simulink model "swhl_arch"  (R2024a)
settings: Solver=FixedStepDiscrete  StartTime=0.0  StopTime=10.0  RelTol=1e-3
undefined symbols (not defined in the file or in its folder): D1, P
settings Model: Creator=Inquisitor  LastModifiedBy=Inquisitor

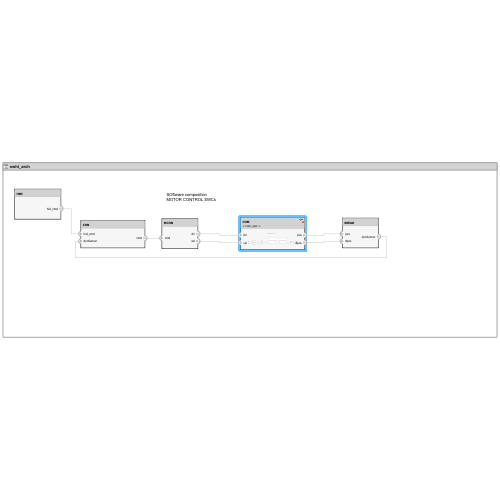
[thumbnail: Simulink's stored preview of the top-level diagram]
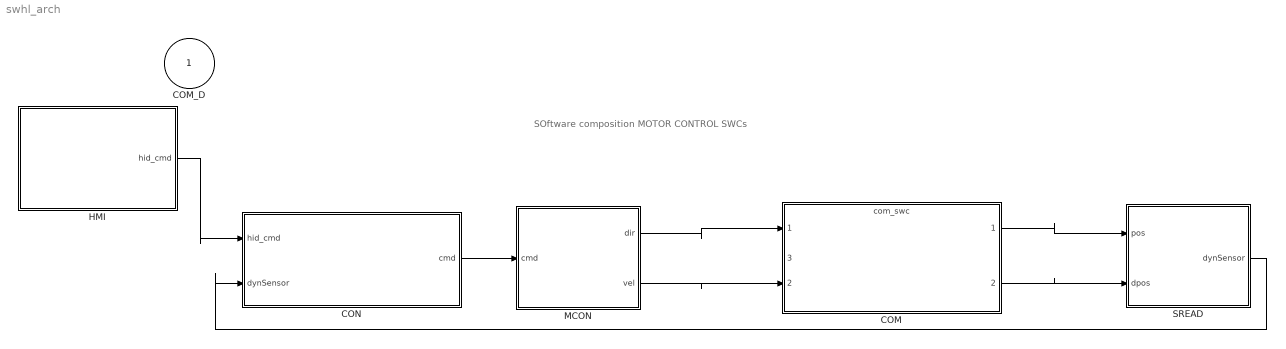
== system swhl_arch ==
  note: SOftware composition
      | MOTOR CONTROL SWCs
  COM_D : Inport  OutputFunctionCall=on
  COM : ModelReference  ModelNameDialog=com_swc.slx  SimulationMode=Normal  ScheduleRates=on  ModelEventPortInfo=P:D1[-2][0][0]  ModelReferenceVersion=1.2
      settings: PortSchema="{\"entries\":[{\"content\":{\"headerSize\":38,\"margin\":15,\"minimumSpacing\":25,\"sides\":[{\"content\":{\"connectorIds\":[\"In1\",\"In2\"]},\"type\":\"ConnectorPlacement.EquallySpacedRectSide\",\"uuid\":\"afd5f5c6-9565-45e0-8f6c-5011a3e66bdb\"},{\"content\":{\"connectorIds\":[\"Out1\",\"Out2\"],\"side\":\"RIGHT\"},\"type\":\"ConnectorPlacement.EquallySpacedRectSide\",\"uuid\":\"137ba84f-98a8-4f32-8497-d281cbf05db7\"},{\"content\":{\"side\":\"TOP\"},\"type\":\"ConnectorPlacement.EquallySpacedRectSide\",\"uuid\":\"8e646a95-539a-43d5-ab96-0f54ad6e94a8\"},{\"content\":{\"connectorIds\":[\"In3\"],\"side\":\"HIDDEN\"},\"type\":\"ConnectorPlacement.EquallySpacedRectSide\",\"uuid\":\"77fa6bc9-fe2f-4392-a70a-4dbebac9b5fe\"}]},\"type\":\"ConnectorPlacement.EquallySpacedConnector\",\"uuid\":\"08e25dfa-be98-4f23-ad10-59dec6d538f8\"}],\"packageUris\":[\"http://schema.mathworks.com/mf0/Connector/R2020b\"],\"version\":\"1.0\"}"
  CON : Subsystem
      settings: PortSchema="{\"entries\":[{\"content\":{\"headerSize\":26,\"margin\":15,\"minimumSpacing\":25,\"sides\":[{\"content\":{\"connectorIds\":[\"In1\",\"In2\"]},\"type\":\"ConnectorPlacement.EquallySpacedRectSide\",\"uuid\":\"afd5f5c6-9565-45e0-8f6c-5011a3e66bdb\"},{\"content\":{\"connectorIds\":[\"Out1\"],\"side\":\"RIGHT\"},\"type\":\"ConnectorPlacement.EquallySpacedRectSide\",\"uuid\":\"137ba84f-98a8-4f32-8497-d281cbf05db7\"},{\"content\":{\"side\":\"TOP\"},\"type\":\"ConnectorPlacement.EquallySpacedRectSide\",\"uuid\":\"8e646a95-539a-43d5-ab96-0f54ad6e94a8\"},{\"content\":{\"side\":\"BOTTOM\"},\"type\":\"ConnectorPlacement.EquallySpacedRectSide\",\"uuid\":\"605cdce3-db15-4b85-b939-147a438ff11d\"}]},\"type\":\"ConnectorPlacement.EquallySpacedConnector\",\"uuid\":\"08e25dfa-be98-4f23-ad10-59dec6d538f8\"}],\"packageUris\":[\"http://schema.mathworks.com/mf0/Connector/R2020b\"],\"version\":\"1.0\"}"
  HMI : Subsystem
      settings: PortSchema="{\"entries\":[{\"content\":{\"headerSize\":26,\"margin\":15,\"minimumSpacing\":25,\"sides\":[{\"content\":{},\"type\":\"ConnectorPlacement.EquallySpacedRectSide\",\"uuid\":\"afd5f5c6-9565-45e0-8f6c-5011a3e66bdb\"},{\"content\":{\"connectorIds\":[\"Out1\"],\"side\":\"RIGHT\"},\"type\":\"ConnectorPlacement.EquallySpacedRectSide\",\"uuid\":\"137ba84f-98a8-4f32-8497-d281cbf05db7\"},{\"content\":{\"side\":\"TOP\"},\"type\":\"ConnectorPlacement.EquallySpacedRectSide\",\"uuid\":\"8e646a95-539a-43d5-ab96-0f54ad6e94a8\"}]},\"type\":\"ConnectorPlacement.EquallySpacedConnector\",\"uuid\":\"08e25dfa-be98-4f23-ad10-59dec6d538f8\"}],\"packageUris\":[\"http://schema.mathworks.com/mf0/Connector/R2020b\"],\"version\":\"1.0\"}"
  MCON : Subsystem
      settings: PortSchema="{\"entries\":[{\"content\":{\"headerSize\":26,\"margin\":15,\"minimumSpacing\":25,\"sides\":[{\"content\":{\"connectorIds\":[\"In1\"]},\"type\":\"ConnectorPlacement.EquallySpacedRectSide\",\"uuid\":\"afd5f5c6-9565-45e0-8f6c-5011a3e66bdb\"},{\"content\":{\"connectorIds\":[\"Out1\",\"Out2\"],\"side\":\"RIGHT\"},\"type\":\"ConnectorPlacement.EquallySpacedRectSide\",\"uuid\":\"137ba84f-98a8-4f32-8497-d281cbf05db7\"},{\"content\":{\"side\":\"TOP\"},\"type\":\"ConnectorPlacement.EquallySpacedRectSide\",\"uuid\":\"8e646a95-539a-43d5-ab96-0f54ad6e94a8\"},{\"content\":{\"side\":\"BOTTOM\"},\"type\":\"ConnectorPlacement.EquallySpacedRectSide\",\"uuid\":\"6073384e-78ac-4ad6-a695-8355c769fbd5\"}]},\"type\":\"ConnectorPlacement.EquallySpacedConnector\",\"uuid\":\"08e25dfa-be98-4f23-ad10-59dec6d538f8\"}],\"packageUris\":[\"http://schema.mathworks.com/mf0/Connector/R2020b\"],\"version\":\"1.0\"}"
  SREAD : Subsystem
      settings: PortSchema="{\"entries\":[{\"content\":{\"headerSize\":26,\"margin\":15,\"minimumSpacing\":25,\"sides\":[{\"content\":{\"connectorIds\":[\"In1\",\"In2\"]},\"type\":\"ConnectorPlacement.EquallySpacedRectSide\",\"uuid\":\"afd5f5c6-9565-45e0-8f6c-5011a3e66bdb\"},{\"content\":{\"connectorIds\":[\"Out1\"],\"side\":\"RIGHT\"},\"type\":\"ConnectorPlacement.EquallySpacedRectSide\",\"uuid\":\"137ba84f-98a8-4f32-8497-d281cbf05db7\"},{\"content\":{\"side\":\"TOP\"},\"type\":\"ConnectorPlacement.EquallySpacedRectSide\",\"uuid\":\"8e646a95-539a-43d5-ab96-0f54ad6e94a8\"}]},\"type\":\"ConnectorPlacement.EquallySpacedConnector\",\"uuid\":\"08e25dfa-be98-4f23-ad10-59dec6d538f8\"}],\"packageUris\":[\"http://schema.mathworks.com/mf0/Connector/R2020b\"],\"version\":\"1.0\"}"
  wires:
  SREAD/1(dynSensor) -> CON/2(dynSensor)
  CON/1(cmd) -> MCON/1(cmd)
  HMI/1(hid_cmd) -> CON/1(hid_cmd)
  MCON/1(dir) -> COM/1
  MCON/2(vel) -> COM/2
  COM/2 -> SREAD/2(dpos)
  COM/1 -> SREAD/1(pos)

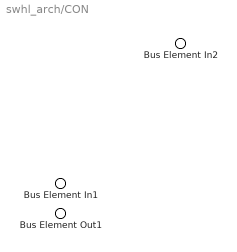
== system swhl_arch/CON ==
  Bus Element In2 : Inport  PortName=hid_cmd
  Bus Element In1 : Inport  Port=2  PortName=dynSensor
  Bus Element Out1 : Outport  PortName=cmd

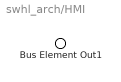
== system swhl_arch/HMI ==
  Bus Element Out1 : Outport  PortName=hid_cmd

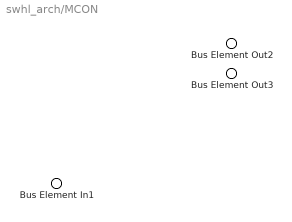
== system swhl_arch/MCON ==
  Bus Element In1 : Inport  PortName=cmd
  Bus Element Out2 : Outport  PortName=dir
  Bus Element Out3 : Outport  Port=2  PortName=vel

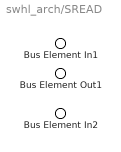
== system swhl_arch/SREAD ==
  Bus Element In1 : Inport  PortName=pos
  Bus Element In2 : Inport  Port=2  PortName=dpos
  Bus Element Out1 : Outport  PortName=dynSensor
